simulink model "festo_proiect"  (R2022b)
settings: Solver=ode45  StartTime=0.0  StopTime=1500  RelTol=1e-3
undefined symbols (not defined in the file): A, C, dqi, hinitial, Hr, Hr1, Hr2, k, k1, k2, k3, k_comp, keta, qinitial, ua
libraries: slpidlib x7
(part 1 of 2)
settings Model: Creator=Alex  LastModifiedBy=Alex

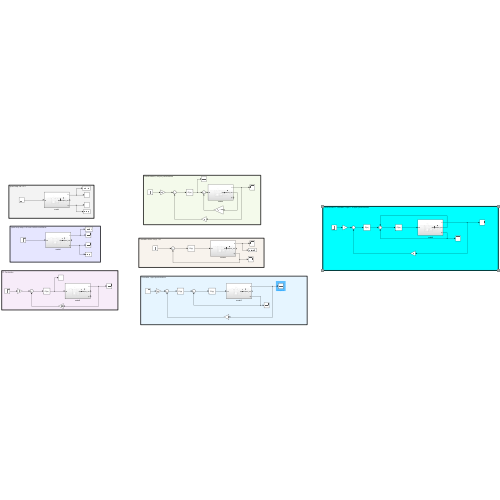
[thumbnail: Simulink's stored preview of the top-level diagram]
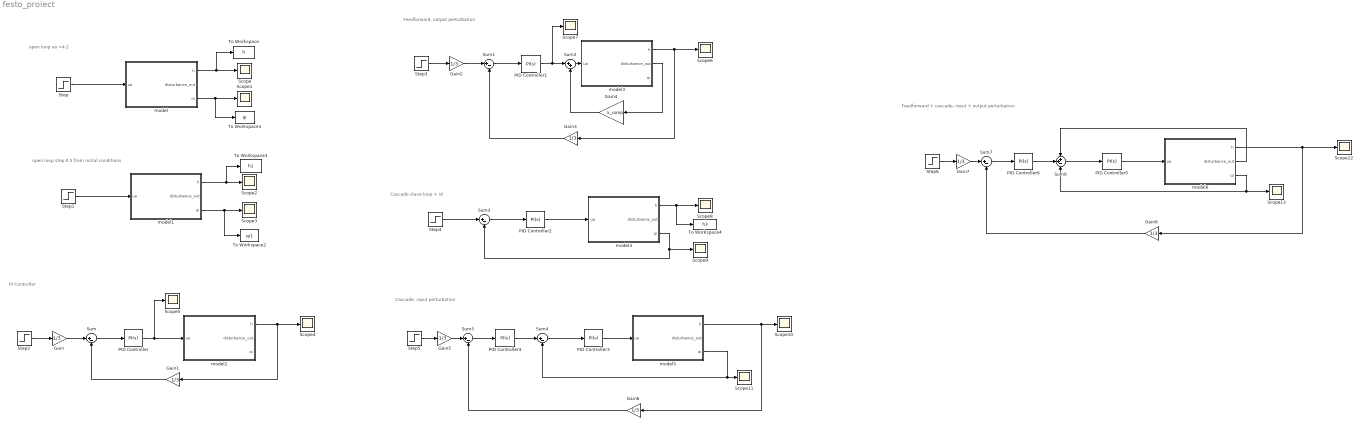
== system festo_proiect ==
  note: Feedforward + cascade, input + output perturbation
  note: Cascade, input perturbation
  note: Cascade slave loop + id
  note: Feedforward, output perturbation
  note: PI Controller
  note: open loop step 0.5 from initial conditions
  note: open loop ua =4.2
  Gain{,1..3,5..8} (8 alike) : Gain  Gain=1/3
  Gain4 : Gain  Gain=k_comp
  PID Controller : slpidlib/PID Controller  Controller=PI  Form=Parallel  TimeDomain=Continuous-time  UseExternalTs=off  SampleTime=-1  IntegratorMethod=Forward Euler  FilterMethod=Forward Euler  ControllerParametersSource=internal  P=Hr.Kp  I=Hr.kp/Hr.Ti  UseKiTs=off  D=0  N=100  UseFilter=on  TunerSelectOption=Transfer Function Based (PID Tuner App)  InitialConditionSource=internal  InitialConditionForIntegrator=ua  InitialConditionForFilter=0  DifferentiatorICPrevScaledInput=0  ExternalReset=none  TrackingMode=off  Kt=1  LimitOutput=off  SatLimitsSource=internal  UpperSaturationLimit=inf  LowerSaturationLimit=-inf  LinearizeAsGain=on  AntiWindupMode=none  Kb=1  LimitIntegrator=off  UpperIntegratorSaturationLimit=inf  LowerIntegratorSaturationLimit=-inf  POutMin=[]  POutMax=[]  IOutMin=[]  IOutMax=[]  DOutMin=[]  DOutMax=[]  NOutMin=[]  NOutMax=[]  SumOutMin=[]  SumOutMax=[]  SaturationOutMin=[]  SaturationOutMax=[]  PParamMin=[]  PParamMax=[]  IParamMin=[]  IParamMax=[]  DParamMin=[]  DParamMax=[]  NParamMin=[]  NParamMax=[]  KbParamMin=[]  KbParamMax=[]  KtParamMin=[]  KtParamMax=[]  KbOutMin=[]  KbOutMax=[]  KtOutMin=[]  KtOutMax=[]  IntegratorOutMin=[]  IntegratorOutMax=[]  FilterOutMin=[]  FilterOutMax=[]  SumI1OutMin=[]  SumI1OutMax=[]  SumI2OutMin=[]  SumI2OutMax=[]  SumI3OutMin=[]  SumI3OutMax=[]  SumI4OutMin=[]  SumI4OutMax=[]  SumDOutMin=[]  SumDOutMax=[]  DifferentiatorOutMin=[]  DifferentiatorOutMax=[]  FilterDiffOutCoefMin=[]  FilterDiffOutCoefMax=[]  ReciprocalOutMin=[]  ReciprocalOutMax=[]  SumDenOutMin=[]  SumDenOutMax=[]  SumNumOutMin=[]  SumNumOutMax=[]  DivideOutMin=[]  DivideOutMax=[]  UdiffTsProdOutMin=[]  UdiffTsProdOutMax=[]  NTsProdOutMin=[]  NTsProdOutMax=[]  UintegralTsProdOutMin=[]  UintegralTsProdOutMax=[]  UngainTsProdOutMin=[]  UngainTsProdOutMax=[]  ClampingZeroOutDataTypeStr=Inherit: Inherit via back propagation  ClampingZeroOutMin=[]  ClampingZeroOutMax=[]  FilterDenConstantOutDataTypeStr=Inherit: Inherit via back propagation  FilterDenConstantOutMin=[]  FilterDenConstantOutMax=[]  PCopyOutDataTypeStr=Inherit: Inherit via back propagation  PCopyOutMin=[]  PCopyOutMax=[]  NCopyOutDataTypeStr=Inherit: Inherit via back propagation  NCopyOutMin=[]  NCopyOutMax=[]  IntegratorContinuousStateAttributes=''  IntegratorStateMustResolveToSignalObject=off  IntegratorRTWStateStorageClass=Auto  FilterContinuousStateAttributes=''  FilterStateMustResolveToSignalObject=off  FilterRTWStateStorageClass=Auto  ParallelPVariant=InternalParameters  IdealPVariant=Disabled  IVariant=InternalParameters  DVariant=Disabled  IntegratorVariant=Continuous  SatVariant=Disabled  AWVariant=Passthrough  PCopyVariant=Disabled  TRVariant=Disabled  FdbkBlocksVariant=Forward  IdealPFdbkVariant=Disabled  SatFdbkVariant=Disabled  DerivativeFilterVariant=Disabled  NVariant=Disabled  NCopyVariant=Disabled_SignalSpec  FilterICVariant=Disabled  IntegratorICVariant=InternalICs  ExternalResetVariant=Disabled  TRSumVariant=Passthrough  SumFdbkVariant=Disabled  SumVariant=Sum_PI  TsampFilterVariant=InternalTs  TsampNgainVariant=Passthrough  TsampIntegralVariant=Passthrough  ExternalSaturationOutDataTypeStr=Inherit: Same as second input
  PID Controller1 : slpidlib/PID Controller  Controller=PI  Form=Parallel  TimeDomain=Continuous-time  UseExternalTs=off  SampleTime=-1  IntegratorMethod=Forward Euler  FilterMethod=Forward Euler  ControllerParametersSource=internal  P=Hr.Kp  I=Hr.kp/Hr.Ti  UseKiTs=off  D=0  N=100  UseFilter=on  TunerSelectOption=Transfer Function Based (PID Tuner App)  InitialConditionSource=internal  InitialConditionForIntegrator=ua  InitialConditionForFilter=0  DifferentiatorICPrevScaledInput=0  ExternalReset=none  TrackingMode=off  Kt=1  LimitOutput=off  SatLimitsSource=internal  UpperSaturationLimit=inf  LowerSaturationLimit=-inf  LinearizeAsGain=on  AntiWindupMode=none  Kb=1  LimitIntegrator=off  UpperIntegratorSaturationLimit=inf  LowerIntegratorSaturationLimit=-inf  POutMin=[]  POutMax=[]  IOutMin=[]  IOutMax=[]  DOutMin=[]  DOutMax=[]  NOutMin=[]  NOutMax=[]  SumOutMin=[]  SumOutMax=[]  SaturationOutMin=[]  SaturationOutMax=[]  PParamMin=[]  PParamMax=[]  IParamMin=[]  IParamMax=[]  DParamMin=[]  DParamMax=[]  NParamMin=[]  NParamMax=[]  KbParamMin=[]  KbParamMax=[]  KtParamMin=[]  KtParamMax=[]  KbOutMin=[]  KbOutMax=[]  KtOutMin=[]  KtOutMax=[]  IntegratorOutMin=[]  IntegratorOutMax=[]  FilterOutMin=[]  FilterOutMax=[]  SumI1OutMin=[]  SumI1OutMax=[]  SumI2OutMin=[]  SumI2OutMax=[]  SumI3OutMin=[]  SumI3OutMax=[]  SumI4OutMin=[]  SumI4OutMax=[]  SumDOutMin=[]  SumDOutMax=[]  DifferentiatorOutMin=[]  DifferentiatorOutMax=[]  FilterDiffOutCoefMin=[]  FilterDiffOutCoefMax=[]  ReciprocalOutMin=[]  ReciprocalOutMax=[]  SumDenOutMin=[]  SumDenOutMax=[]  SumNumOutMin=[]  SumNumOutMax=[]  DivideOutMin=[]  DivideOutMax=[]  UdiffTsProdOutMin=[]  UdiffTsProdOutMax=[]  NTsProdOutMin=[]  NTsProdOutMax=[]  UintegralTsProdOutMin=[]  UintegralTsProdOutMax=[]  UngainTsProdOutMin=[]  UngainTsProdOutMax=[]  ClampingZeroOutDataTypeStr=Inherit: Inherit via back propagation  ClampingZeroOutMin=[]  ClampingZeroOutMax=[]  FilterDenConstantOutDataTypeStr=Inherit: Inherit via back propagation  FilterDenConstantOutMin=[]  FilterDenConstantOutMax=[]  PCopyOutDataTypeStr=Inherit: Inherit via back propagation  PCopyOutMin=[]  PCopyOutMax=[]  NCopyOutDataTypeStr=Inherit: Inherit via back propagation  NCopyOutMin=[]  NCopyOutMax=[]  IntegratorContinuousStateAttributes=''  IntegratorStateMustResolveToSignalObject=off  IntegratorRTWStateStorageClass=Auto  FilterContinuousStateAttributes=''  FilterStateMustResolveToSignalObject=off  FilterRTWStateStorageClass=Auto  ParallelPVariant=InternalParameters  IdealPVariant=Disabled  IVariant=InternalParameters  DVariant=Disabled  IntegratorVariant=Continuous  SatVariant=Disabled  AWVariant=Passthrough  PCopyVariant=Disabled  TRVariant=Disabled  FdbkBlocksVariant=Forward  IdealPFdbkVariant=Disabled  SatFdbkVariant=Disabled  DerivativeFilterVariant=Disabled  NVariant=Disabled  NCopyVariant=Disabled_SignalSpec  FilterICVariant=Disabled  IntegratorICVariant=InternalICs  ExternalResetVariant=Disabled  TRSumVariant=Passthrough  SumFdbkVariant=Disabled  SumVariant=Sum_PI  TsampFilterVariant=InternalTs  TsampNgainVariant=Passthrough  TsampIntegralVariant=Passthrough  ExternalSaturationOutDataTypeStr=Inherit: Same as second input
  PID Controller2 : slpidlib/PID Controller  Controller=PI  Form=Parallel  TimeDomain=Continuous-time  UseExternalTs=off  SampleTime=-1  IntegratorMethod=Forward Euler  FilterMethod=Forward Euler  ControllerParametersSource=internal  P=Hr1.Kp  I=Hr1.Kp/Hr1.Ti  UseKiTs=off  D=0  N=100  UseFilter=on  TunerSelectOption=Transfer Function Based (PID Tuner App)  InitialConditionSource=internal  InitialConditionForIntegrator=ua  InitialConditionForFilter=0  DifferentiatorICPrevScaledInput=0  ExternalReset=none  TrackingMode=off  Kt=1  LimitOutput=off  SatLimitsSource=internal  UpperSaturationLimit=inf  LowerSaturationLimit=-inf  LinearizeAsGain=on  AntiWindupMode=none  Kb=1  LimitIntegrator=off  UpperIntegratorSaturationLimit=inf  LowerIntegratorSaturationLimit=-inf  POutMin=[]  POutMax=[]  IOutMin=[]  IOutMax=[]  DOutMin=[]  DOutMax=[]  NOutMin=[]  NOutMax=[]  SumOutMin=[]  SumOutMax=[]  SaturationOutMin=[]  SaturationOutMax=[]  PParamMin=[]  PParamMax=[]  IParamMin=[]  IParamMax=[]  DParamMin=[]  DParamMax=[]  NParamMin=[]  NParamMax=[]  KbParamMin=[]  KbParamMax=[]  KtParamMin=[]  KtParamMax=[]  KbOutMin=[]  KbOutMax=[]  KtOutMin=[]  KtOutMax=[]  IntegratorOutMin=[]  IntegratorOutMax=[]  FilterOutMin=[]  FilterOutMax=[]  SumI1OutMin=[]  SumI1OutMax=[]  SumI2OutMin=[]  SumI2OutMax=[]  SumI3OutMin=[]  SumI3OutMax=[]  SumI4OutMin=[]  SumI4OutMax=[]  SumDOutMin=[]  SumDOutMax=[]  DifferentiatorOutMin=[]  DifferentiatorOutMax=[]  FilterDiffOutCoefMin=[]  FilterDiffOutCoefMax=[]  ReciprocalOutMin=[]  ReciprocalOutMax=[]  SumDenOutMin=[]  SumDenOutMax=[]  SumNumOutMin=[]  SumNumOutMax=[]  DivideOutMin=[]  DivideOutMax=[]  UdiffTsProdOutMin=[]  UdiffTsProdOutMax=[]  NTsProdOutMin=[]  NTsProdOutMax=[]  UintegralTsProdOutMin=[]  UintegralTsProdOutMax=[]  UngainTsProdOutMin=[]  UngainTsProdOutMax=[]  ClampingZeroOutDataTypeStr=Inherit: Inherit via back propagation  ClampingZeroOutMin=[]  ClampingZeroOutMax=[]  FilterDenConstantOutDataTypeStr=Inherit: Inherit via back propagation  FilterDenConstantOutMin=[]  FilterDenConstantOutMax=[]  PCopyOutDataTypeStr=Inherit: Inherit via back propagation  PCopyOutMin=[]  PCopyOutMax=[]  NCopyOutDataTypeStr=Inherit: Inherit via back propagation  NCopyOutMin=[]  NCopyOutMax=[]  IntegratorContinuousStateAttributes=''  IntegratorStateMustResolveToSignalObject=off  IntegratorRTWStateStorageClass=Auto  FilterContinuousStateAttributes=''  FilterStateMustResolveToSignalObject=off  FilterRTWStateStorageClass=Auto  ParallelPVariant=InternalParameters  IdealPVariant=Disabled  IVariant=InternalParameters  DVariant=Disabled  IntegratorVariant=Continuous  SatVariant=Disabled  AWVariant=Passthrough  PCopyVariant=Disabled  TRVariant=Disabled  FdbkBlocksVariant=Forward  IdealPFdbkVariant=Disabled  SatFdbkVariant=Disabled  DerivativeFilterVariant=Disabled  NVariant=Disabled  NCopyVariant=Disabled_SignalSpec  FilterICVariant=Disabled  IntegratorICVariant=InternalICs  ExternalResetVariant=Disabled  TRSumVariant=Passthrough  SumFdbkVariant=Disabled  SumVariant=Sum_PI  TsampFilterVariant=InternalTs  TsampNgainVariant=Passthrough  TsampIntegralVariant=Passthrough  ExternalSaturationOutDataTypeStr=Inherit: Same as second input
  PID Controller3 : slpidlib/PID Controller  Controller=PI  Form=Parallel  TimeDomain=Continuous-time  UseExternalTs=off  SampleTime=-1  IntegratorMethod=Forward Euler  FilterMethod=Forward Euler  ControllerParametersSource=internal  P=Hr1.Kp  I=Hr1.Kp/Hr1.Ti  UseKiTs=off  D=0  N=100  UseFilter=on  TunerSelectOption=Transfer Function Based (PID Tuner App)  InitialConditionSource=internal  InitialConditionForIntegrator=ua  InitialConditionForFilter=0  DifferentiatorICPrevScaledInput=0  ExternalReset=none  TrackingMode=off  Kt=1  LimitOutput=off  SatLimitsSource=internal  UpperSaturationLimit=inf  LowerSaturationLimit=-inf  LinearizeAsGain=on  AntiWindupMode=none  Kb=1  LimitIntegrator=off  UpperIntegratorSaturationLimit=inf  LowerIntegratorSaturationLimit=-inf  POutMin=[]  POutMax=[]  IOutMin=[]  IOutMax=[]  DOutMin=[]  DOutMax=[]  NOutMin=[]  NOutMax=[]  SumOutMin=[]  SumOutMax=[]  SaturationOutMin=[]  SaturationOutMax=[]  PParamMin=[]  PParamMax=[]  IParamMin=[]  IParamMax=[]  DParamMin=[]  DParamMax=[]  NParamMin=[]  NParamMax=[]  KbParamMin=[]  KbParamMax=[]  KtParamMin=[]  KtParamMax=[]  KbOutMin=[]  KbOutMax=[]  KtOutMin=[]  KtOutMax=[]  IntegratorOutMin=[]  IntegratorOutMax=[]  FilterOutMin=[]  FilterOutMax=[]  SumI1OutMin=[]  SumI1OutMax=[]  SumI2OutMin=[]  SumI2OutMax=[]  SumI3OutMin=[]  SumI3OutMax=[]  SumI4OutMin=[]  SumI4OutMax=[]  SumDOutMin=[]  SumDOutMax=[]  DifferentiatorOutMin=[]  DifferentiatorOutMax=[]  FilterDiffOutCoefMin=[]  FilterDiffOutCoefMax=[]  ReciprocalOutMin=[]  ReciprocalOutMax=[]  SumDenOutMin=[]  SumDenOutMax=[]  SumNumOutMin=[]  SumNumOutMax=[]  DivideOutMin=[]  DivideOutMax=[]  UdiffTsProdOutMin=[]  UdiffTsProdOutMax=[]  NTsProdOutMin=[]  NTsProdOutMax=[]  UintegralTsProdOutMin=[]  UintegralTsProdOutMax=[]  UngainTsProdOutMin=[]  UngainTsProdOutMax=[]  ClampingZeroOutDataTypeStr=Inherit: Inherit via back propagation  ClampingZeroOutMin=[]  ClampingZeroOutMax=[]  FilterDenConstantOutDataTypeStr=Inherit: Inherit via back propagation  FilterDenConstantOutMin=[]  FilterDenConstantOutMax=[]  PCopyOutDataTypeStr=Inherit: Inherit via back propagation  PCopyOutMin=[]  PCopyOutMax=[]  NCopyOutDataTypeStr=Inherit: Inherit via back propagation  NCopyOutMin=[]  NCopyOutMax=[]  IntegratorContinuousStateAttributes=''  IntegratorStateMustResolveToSignalObject=off  IntegratorRTWStateStorageClass=Auto  FilterContinuousStateAttributes=''  FilterStateMustResolveToSignalObject=off  FilterRTWStateStorageClass=Auto  ParallelPVariant=InternalParameters  IdealPVariant=Disabled  IVariant=InternalParameters  DVariant=Disabled  IntegratorVariant=Continuous  SatVariant=Disabled  AWVariant=Passthrough  PCopyVariant=Disabled  TRVariant=Disabled  FdbkBlocksVariant=Forward  IdealPFdbkVariant=Disabled  SatFdbkVariant=Disabled  DerivativeFilterVariant=Disabled  NVariant=Disabled  NCopyVariant=Disabled_SignalSpec  FilterICVariant=Disabled  IntegratorICVariant=InternalICs  ExternalResetVariant=Disabled  TRSumVariant=Passthrough  SumFdbkVariant=Disabled  SumVariant=Sum_PI  TsampFilterVariant=InternalTs  TsampNgainVariant=Passthrough  TsampIntegralVariant=Passthrough  ExternalSaturationOutDataTypeStr=Inherit: Same as second input
  PID Controller4 : slpidlib/PID Controller  Controller=PI  Form=Parallel  TimeDomain=Continuous-time  UseExternalTs=off  SampleTime=-1  IntegratorMethod=Forward Euler  FilterMethod=Forward Euler  ControllerParametersSource=internal  P=Hr2.Kp  I=Hr2.Kp/Hr2.Ti  UseKiTs=off  D=0  N=100  UseFilter=on  TunerSelectOption=Transfer Function Based (PID Tuner App)  InitialConditionSource=internal  InitialConditionForIntegrator=qinitial  InitialConditionForFilter=0  DifferentiatorICPrevScaledInput=0  ExternalReset=none  TrackingMode=off  Kt=1  LimitOutput=off  SatLimitsSource=internal  UpperSaturationLimit=inf  LowerSaturationLimit=-inf  LinearizeAsGain=on  AntiWindupMode=none  Kb=1  LimitIntegrator=off  UpperIntegratorSaturationLimit=inf  LowerIntegratorSaturationLimit=-inf  POutMin=[]  POutMax=[]  IOutMin=[]  IOutMax=[]  DOutMin=[]  DOutMax=[]  NOutMin=[]  NOutMax=[]  SumOutMin=[]  SumOutMax=[]  SaturationOutMin=[]  SaturationOutMax=[]  PParamMin=[]  PParamMax=[]  IParamMin=[]  IParamMax=[]  DParamMin=[]  DParamMax=[]  NParamMin=[]  NParamMax=[]  KbParamMin=[]  KbParamMax=[]  KtParamMin=[]  KtParamMax=[]  KbOutMin=[]  KbOutMax=[]  KtOutMin=[]  KtOutMax=[]  IntegratorOutMin=[]  IntegratorOutMax=[]  FilterOutMin=[]  FilterOutMax=[]  SumI1OutMin=[]  SumI1OutMax=[]  SumI2OutMin=[]  SumI2OutMax=[]  SumI3OutMin=[]  SumI3OutMax=[]  SumI4OutMin=[]  SumI4OutMax=[]  SumDOutMin=[]  SumDOutMax=[]  DifferentiatorOutMin=[]  DifferentiatorOutMax=[]  FilterDiffOutCoefMin=[]  FilterDiffOutCoefMax=[]  ReciprocalOutMin=[]  ReciprocalOutMax=[]  SumDenOutMin=[]  SumDenOutMax=[]  SumNumOutMin=[]  SumNumOutMax=[]  DivideOutMin=[]  DivideOutMax=[]  UdiffTsProdOutMin=[]  UdiffTsProdOutMax=[]  NTsProdOutMin=[]  NTsProdOutMax=[]  UintegralTsProdOutMin=[]  UintegralTsProdOutMax=[]  UngainTsProdOutMin=[]  UngainTsProdOutMax=[]  ClampingZeroOutDataTypeStr=Inherit: Inherit via back propagation  ClampingZeroOutMin=[]  ClampingZeroOutMax=[]  FilterDenConstantOutDataTypeStr=Inherit: Inherit via back propagation  FilterDenConstantOutMin=[]  FilterDenConstantOutMax=[]  PCopyOutDataTypeStr=Inherit: Inherit via back propagation  PCopyOutMin=[]  PCopyOutMax=[]  NCopyOutDataTypeStr=Inherit: Inherit via back propagation  NCopyOutMin=[]  NCopyOutMax=[]  IntegratorContinuousStateAttributes=''  IntegratorStateMustResolveToSignalObject=off  IntegratorRTWStateStorageClass=Auto  FilterContinuousStateAttributes=''  FilterStateMustResolveToSignalObject=off  FilterRTWStateStorageClass=Auto  ParallelPVariant=InternalParameters  IdealPVariant=Disabled  IVariant=InternalParameters  DVariant=Disabled  IntegratorVariant=Continuous  SatVariant=Disabled  AWVariant=Passthrough  PCopyVariant=Disabled  TRVariant=Disabled  FdbkBlocksVariant=Forward  IdealPFdbkVariant=Disabled  SatFdbkVariant=Disabled  DerivativeFilterVariant=Disabled  NVariant=Disabled  NCopyVariant=Disabled_SignalSpec  FilterICVariant=Disabled  IntegratorICVariant=InternalICs  ExternalResetVariant=Disabled  TRSumVariant=Passthrough  SumFdbkVariant=Disabled  SumVariant=Sum_PI  TsampFilterVariant=InternalTs  TsampNgainVariant=Passthrough  TsampIntegralVariant=Passthrough  ExternalSaturationOutDataTypeStr=Inherit: Same as second input
  PID Controller5 : slpidlib/PID Controller  Controller=PI  Form=Parallel  TimeDomain=Continuous-time  UseExternalTs=off  SampleTime=-1  IntegratorMethod=Forward Euler  FilterMethod=Forward Euler  ControllerParametersSource=internal  P=Hr1.Kp  I=Hr1.Kp/Hr1.Ti  UseKiTs=off  D=0  N=100  UseFilter=on  TunerSelectOption=Transfer Function Based (PID Tuner App)  InitialConditionSource=internal  InitialConditionForIntegrator=ua  InitialConditionForFilter=0  DifferentiatorICPrevScaledInput=0  ExternalReset=none  TrackingMode=off  Kt=1  LimitOutput=off  SatLimitsSource=internal  UpperSaturationLimit=inf  LowerSaturationLimit=-inf  LinearizeAsGain=on  AntiWindupMode=none  Kb=1  LimitIntegrator=off  UpperIntegratorSaturationLimit=inf  LowerIntegratorSaturationLimit=-inf  POutMin=[]  POutMax=[]  IOutMin=[]  IOutMax=[]  DOutMin=[]  DOutMax=[]  NOutMin=[]  NOutMax=[]  SumOutMin=[]  SumOutMax=[]  SaturationOutMin=[]  SaturationOutMax=[]  PParamMin=[]  PParamMax=[]  IParamMin=[]  IParamMax=[]  DParamMin=[]  DParamMax=[]  NParamMin=[]  NParamMax=[]  KbParamMin=[]  KbParamMax=[]  KtParamMin=[]  KtParamMax=[]  KbOutMin=[]  KbOutMax=[]  KtOutMin=[]  KtOutMax=[]  IntegratorOutMin=[]  IntegratorOutMax=[]  FilterOutMin=[]  FilterOutMax=[]  SumI1OutMin=[]  SumI1OutMax=[]  SumI2OutMin=[]  SumI2OutMax=[]  SumI3OutMin=[]  SumI3OutMax=[]  SumI4OutMin=[]  SumI4OutMax=[]  SumDOutMin=[]  SumDOutMax=[]  DifferentiatorOutMin=[]  DifferentiatorOutMax=[]  FilterDiffOutCoefMin=[]  FilterDiffOutCoefMax=[]  ReciprocalOutMin=[]  ReciprocalOutMax=[]  SumDenOutMin=[]  SumDenOutMax=[]  SumNumOutMin=[]  SumNumOutMax=[]  DivideOutMin=[]  DivideOutMax=[]  UdiffTsProdOutMin=[]  UdiffTsProdOutMax=[]  NTsProdOutMin=[]  NTsProdOutMax=[]  UintegralTsProdOutMin=[]  UintegralTsProdOutMax=[]  UngainTsProdOutMin=[]  UngainTsProdOutMax=[]  ClampingZeroOutDataTypeStr=Inherit: Inherit via back propagation  ClampingZeroOutMin=[]  ClampingZeroOutMax=[]  FilterDenConstantOutDataTypeStr=Inherit: Inherit via back propagation  FilterDenConstantOutMin=[]  FilterDenConstantOutMax=[]  PCopyOutDataTypeStr=Inherit: Inherit via back propagation  PCopyOutMin=[]  PCopyOutMax=[]  NCopyOutDataTypeStr=Inherit: Inherit via back propagation  NCopyOutMin=[]  NCopyOutMax=[]  IntegratorContinuousStateAttributes=''  IntegratorStateMustResolveToSignalObject=off  IntegratorRTWStateStorageClass=Auto  FilterContinuousStateAttributes=''  FilterStateMustResolveToSignalObject=off  FilterRTWStateStorageClass=Auto  ParallelPVariant=InternalParameters  IdealPVariant=Disabled  IVariant=InternalParameters  DVariant=Disabled  IntegratorVariant=Continuous  SatVariant=Disabled  AWVariant=Passthrough  PCopyVariant=Disabled  TRVariant=Disabled  FdbkBlocksVariant=Forward  IdealPFdbkVariant=Disabled  SatFdbkVariant=Disabled  DerivativeFilterVariant=Disabled  NVariant=Disabled  NCopyVariant=Disabled_SignalSpec  FilterICVariant=Disabled  IntegratorICVariant=InternalICs  ExternalResetVariant=Disabled  TRSumVariant=Passthrough  SumFdbkVariant=Disabled  SumVariant=Sum_PI  TsampFilterVariant=InternalTs  TsampNgainVariant=Passthrough  TsampIntegralVariant=Passthrough  ExternalSaturationOutDataTypeStr=Inherit: Same as second input
  PID Controller6 : slpidlib/PID Controller  Controller=PI  Form=Parallel  TimeDomain=Continuous-time  UseExternalTs=off  SampleTime=-1  IntegratorMethod=Forward Euler  FilterMethod=Forward Euler  ControllerParametersSource=internal  P=Hr2.Kp  I=Hr2.Kp/Hr2.Ti  UseKiTs=off  D=0  N=100  UseFilter=on  TunerSelectOption=Transfer Function Based (PID Tuner App)  InitialConditionSource=internal  InitialConditionForIntegrator=qinitial  InitialConditionForFilter=0  DifferentiatorICPrevScaledInput=0  ExternalReset=none  TrackingMode=off  Kt=1  LimitOutput=off  SatLimitsSource=internal  UpperSaturationLimit=inf  LowerSaturationLimit=-inf  LinearizeAsGain=on  AntiWindupMode=none  Kb=1  LimitIntegrator=off  UpperIntegratorSaturationLimit=inf  LowerIntegratorSaturationLimit=-inf  POutMin=[]  POutMax=[]  IOutMin=[]  IOutMax=[]  DOutMin=[]  DOutMax=[]  NOutMin=[]  NOutMax=[]  SumOutMin=[]  SumOutMax=[]  SaturationOutMin=[]  SaturationOutMax=[]  PParamMin=[]  PParamMax=[]  IParamMin=[]  IParamMax=[]  DParamMin=[]  DParamMax=[]  NParamMin=[]  NParamMax=[]  KbParamMin=[]  KbParamMax=[]  KtParamMin=[]  KtParamMax=[]  KbOutMin=[]  KbOutMax=[]  KtOutMin=[]  KtOutMax=[]  IntegratorOutMin=[]  IntegratorOutMax=[]  FilterOutMin=[]  FilterOutMax=[]  SumI1OutMin=[]  SumI1OutMax=[]  SumI2OutMin=[]  SumI2OutMax=[]  SumI3OutMin=[]  SumI3OutMax=[]  SumI4OutMin=[]  SumI4OutMax=[]  SumDOutMin=[]  SumDOutMax=[]  DifferentiatorOutMin=[]  DifferentiatorOutMax=[]  FilterDiffOutCoefMin=[]  FilterDiffOutCoefMax=[]  ReciprocalOutMin=[]  ReciprocalOutMax=[]  SumDenOutMin=[]  SumDenOutMax=[]  SumNumOutMin=[]  SumNumOutMax=[]  DivideOutMin=[]  DivideOutMax=[]  UdiffTsProdOutMin=[]  UdiffTsProdOutMax=[]  NTsProdOutMin=[]  NTsProdOutMax=[]  UintegralTsProdOutMin=[]  UintegralTsProdOutMax=[]  UngainTsProdOutMin=[]  UngainTsProdOutMax=[]  ClampingZeroOutDataTypeStr=Inherit: Inherit via back propagation  ClampingZeroOutMin=[]  ClampingZeroOutMax=[]  FilterDenConstantOutDataTypeStr=Inherit: Inherit via back propagation  FilterDenConstantOutMin=[]  FilterDenConstantOutMax=[]  PCopyOutDataTypeStr=Inherit: Inherit via back propagation  PCopyOutMin=[]  PCopyOutMax=[]  NCopyOutDataTypeStr=Inherit: Inherit via back propagation  NCopyOutMin=[]  NCopyOutMax=[]  IntegratorContinuousStateAttributes=''  IntegratorStateMustResolveToSignalObject=off  IntegratorRTWStateStorageClass=Auto  FilterContinuousStateAttributes=''  FilterStateMustResolveToSignalObject=off  FilterRTWStateStorageClass=Auto  ParallelPVariant=InternalParameters  IdealPVariant=Disabled  IVariant=InternalParameters  DVariant=Disabled  IntegratorVariant=Continuous  SatVariant=Disabled  AWVariant=Passthrough  PCopyVariant=Disabled  TRVariant=Disabled  FdbkBlocksVariant=Forward  IdealPFdbkVariant=Disabled  SatFdbkVariant=Disabled  DerivativeFilterVariant=Disabled  NVariant=Disabled  NCopyVariant=Disabled_SignalSpec  FilterICVariant=Disabled  IntegratorICVariant=InternalICs  ExternalResetVariant=Disabled  TRSumVariant=Passthrough  SumFdbkVariant=Disabled  SumVariant=Sum_PI  TsampFilterVariant=InternalTs  TsampNgainVariant=Passthrough  TsampIntegralVariant=Passthrough  ExternalSaturationOutDataTypeStr=Inherit: Same as second input
  Scope{,1..13} (14 alike) : Scope
  Step : Step  Time=0  After=ua  SampleTime=0
  Step1 : Step  Time=0  Before=ua  After=ua+0.5  SampleTime=0
  Step{2..3,5..6} (4 alike) : Step  Time=0  Before=hinitial  After=13  SampleTime=0
  Step4 : Step  Time=0  Before=qinitial  After=qinitial+dqi  SampleTime=0
  Sum{,1,3..5,7} (6 alike) : Sum  Inputs=|+-
  Sum2 : Sum  Inputs=|++
  Sum6 : Sum  Inputs=++-
  To Workspace : ToWorkspace  VariableName=h  SampleTime=-1
  To Workspace1 : ToWorkspace  VariableName=qi  SampleTime=-1
  To Workspace2 : ToWorkspace  VariableName=qi1  SampleTime=-1
  To Workspace3 : ToWorkspace  VariableName=h1  SampleTime=-1
  To Workspace4 : ToWorkspace  VariableName=h3  SampleTime=-1
  model : Subsystem
  model1 : Subsystem
  model2 : Subsystem
  model3 : Subsystem
  model4 : Subsystem
  model5 : Subsystem
  model6 : Subsystem
  wires:
  Step/1 -> model/1(ua)
  model/1(h) -> To Workspace/1, Scope/1
  model/3(qi) -> To Workspace1/1, Scope1/1
  Step1/1 -> model1/1(ua)
  model1/3(qi) -> To Workspace2/1, Scope3/1
  model1/1(h) -> To Workspace3/1, Scope2/1
  model2/1(h) -> Scope4/1, Gain1/1
  PID Controller/1 -> Scope5/1, model2/1(ua)
  Sum/1 -> PID Controller/1
  Gain/1 -> Sum/1
  Step2/1 -> Gain/1
  Gain1/1 -> Sum/2
  Gain3/1 -> Sum1/2
  Step3/1 -> Gain2/1
  Gain2/1 -> Sum1/1
  Sum1/1 -> PID Controller1/1
  PID Controller1/1 -> Sum2/1, Scope7/1
  model3/1(h) -> Gain3/1, Scope6/1
  Sum2/1 -> model3/1(ua)
  model3/2(disturbance_out) -> Gain4/1
  Gain4/1 -> Sum2/2
  model4/1(h) -> To Workspace4/1, Scope8/1
  PID Controller2/1 -> model4/1(ua)
  Sum3/1 -> PID Controller2/1
  model4/3(qi) -> Scope9/1, Sum3/2
  Step4/1 -> Sum3/1
  model5/3(qi) -> Sum4/2, Scope11/1
  Sum4/1 -> PID Controller3/1
  PID Controller3/1 -> model5/1(ua)
  model5/1(h) -> Scope10/1, Gain6/1
  PID Controller4/1 -> Sum4/1
  Step5/1 -> Gain5/1
  Sum5/1 -> PID Controller4/1
  Gain5/1 -> Sum5/1
  Gain6/1 -> Sum5/2
  Gain8/1 -> Sum7/2
  Gain7/1 -> Sum7/1
  Sum7/1 -> PID Controller6/1
  Step6/1 -> Gain7/1
  PID Controller6/1 -> Sum6/2
  model6/1(h) -> Gain8/1, Scope12/1
  PID Controller5/1 -> model6/1(ua)
  Sum6/1 -> PID Controller5/1
  model6/3(qi) -> Sum6/3, Scope13/1
  model6/2(disturbance_out) -> Sum6/1

== system festo_proiect/model ==
  ua : Inport
  Amplificator : Subsystem
  Curent rotoric : Subsystem
  Filtru : Subsystem
  Motor : Subsystem
  Pompa : Subsystem
  Randament pompa : Subsystem
  Rezervor : Subsystem
  disturbance_in : Step  Commented=on  Time=250  After=0.1*k  SampleTime=0
  h : Outport
  disturbance_out : Outport  Port=2
  qi : Outport  Port=3
  wires:
  Randament pompa/1(eta) -> Curent rotoric/2(eta)
  Rezervor/1(h) -> h/1, Pompa/2(h), Curent rotoric/3(h)
  Amplificator/1(um) -> Curent rotoric/4(um), Randament pompa/2(um), Motor/1(um)
  Motor/1(km*n) -> Pompa/1(km*n)
  ua/1 -> Amplificator/1(ua)
  Curent rotoric/1(im) -> Motor/2(im)
  Pompa/1(q) -> Filtru/1(q)
  Filtru/1(q_f) -> Rezervor/1(q), qi/1, Curent rotoric/1(q), Randament pompa/1(q)
  disturbance_in/1 -> Pompa/3(perturbatie k)
  Rezervor/2(disturbance_out) -> disturbance_out/1

== system festo_proiect/model1 ==
  ua : Inport
  Amplificator : Subsystem
  Curent rotoric : Subsystem
  Filtru : Subsystem
  Motor : Subsystem
  Pompa : Subsystem
  Randament pompa : Subsystem
  Rezervor : Subsystem
  disturbance_in : Step  Commented=on  Time=250  After=0.1*k  SampleTime=0
  h : Outport
  disturbance_out : Outport  Port=2
  qi : Outport  Port=3
  wires:
  Rezervor/2(disturbance_out) -> disturbance_out/1
  disturbance_in/1 -> Pompa/3(perturbatie k)
  Filtru/1(q_f) -> Randament pompa/1(q), Curent rotoric/1(q), qi/1, Rezervor/1(q)
  Pompa/1(q) -> Filtru/1(q)
  Curent rotoric/1(im) -> Motor/2(im)
  ua/1 -> Amplificator/1(ua)
  Motor/1(km*n) -> Pompa/1(km*n)
  Amplificator/1(um) -> Motor/1(um), Randament pompa/2(um), Curent rotoric/4(um)
  Rezervor/1(h) -> Curent rotoric/3(h), Pompa/2(h), h/1
  Randament pompa/1(eta) -> Curent rotoric/2(eta)

== system festo_proiect/model2 ==
  ua : Inport
  Amplificator : Subsystem
  Curent rotoric : Subsystem
  Filtru : Subsystem
  Motor : Subsystem
  Pompa : Subsystem
  Randament pompa : Subsystem
  Rezervor : Subsystem
  disturbance_in : Step  Commented=on  Time=250  After=0.1*k  SampleTime=0
  h : Outport
  disturbance_out : Outport  Port=2
  qi : Outport  Port=3
  wires:
  Randament pompa/1(eta) -> Curent rotoric/2(eta)
  Rezervor/1(h) -> h/1, Pompa/2(h), Curent rotoric/3(h)
  Amplificator/1(um) -> Curent rotoric/4(um), Randament pompa/2(um), Motor/1(um)
  Motor/1(km*n) -> Pompa/1(km*n)
  ua/1 -> Amplificator/1(ua)
  Curent rotoric/1(im) -> Motor/2(im)
  Pompa/1(q) -> Filtru/1(q)
  Filtru/1(q_f) -> Rezervor/1(q), qi/1, Curent rotoric/1(q), Randament pompa/1(q)
  disturbance_in/1 -> Pompa/3(perturbatie k)
  Rezervor/2(disturbance_out) -> disturbance_out/1

== system festo_proiect/model3 ==
  ua : Inport
  Amplificator : Subsystem
  Curent rotoric : Subsystem
  Filtru : Subsystem
  Motor : Subsystem
  Pompa : Subsystem
  Randament pompa : Subsystem
  Rezervor : Subsystem
  disturbance_in : Step  Commented=on  Time=250  After=0.1*k  SampleTime=0
  h : Outport
  disturbance_out : Outport  Port=2
  qi : Outport  Port=3
  wires:
  Rezervor/2(disturbance_out) -> disturbance_out/1
  disturbance_in/1 -> Pompa/3(perturbatie k)
  Filtru/1(q_f) -> Randament pompa/1(q), Curent rotoric/1(q), qi/1, Rezervor/1(q)
  Pompa/1(q) -> Filtru/1(q)
  Curent rotoric/1(im) -> Motor/2(im)
  ua/1 -> Amplificator/1(ua)
  Motor/1(km*n) -> Pompa/1(km*n)
  Amplificator/1(um) -> Motor/1(um), Randament pompa/2(um), Curent rotoric/4(um)
  Rezervor/1(h) -> Curent rotoric/3(h), Pompa/2(h), h/1
  Randament pompa/1(eta) -> Curent rotoric/2(eta)

== system festo_proiect/model4 ==
  ua : Inport
  Amplificator : Subsystem
  Curent rotoric : Subsystem
  Filtru : Subsystem
  Motor : Subsystem
  Pompa : Subsystem
  Randament pompa : Subsystem
  Rezervor : Subsystem
  disturbance_in : Step  Commented=on  Time=250  After=0.1*k  SampleTime=0
  h : Outport
  disturbance_out : Outport  Port=2
  qi : Outport  Port=3
  wires:
  Randament pompa/1(eta) -> Curent rotoric/2(eta)
  Rezervor/1(h) -> h/1, Pompa/2(h), Curent rotoric/3(h)
  Amplificator/1(um) -> Curent rotoric/4(um), Randament pompa/2(um), Motor/1(um)
  Motor/1(km*n) -> Pompa/1(km*n)
  ua/1 -> Amplificator/1(ua)
  Curent rotoric/1(im) -> Motor/2(im)
  Pompa/1(q) -> Filtru/1(q)
  Filtru/1(q_f) -> Rezervor/1(q), qi/1, Curent rotoric/1(q), Randament pompa/1(q)
  disturbance_in/1 -> Pompa/3(perturbatie k)
  Rezervor/2(disturbance_out) -> disturbance_out/1

== system festo_proiect/model5 ==
  ua : Inport
  Amplificator : Subsystem
  Curent rotoric : Subsystem
  Filtru : Subsystem
  Motor : Subsystem
  Pompa : Subsystem
  Randament pompa : Subsystem
  Rezervor : Subsystem
  disturbance_in : Step  Time=250  After=0.1*k  SampleTime=0
  h : Outport
  disturbance_out : Outport  Port=2
  qi : Outport  Port=3
  wires:
  Rezervor/2(disturbance_out) -> disturbance_out/1
  disturbance_in/1 -> Pompa/3(perturbatie k)
  Filtru/1(q_f) -> Randament pompa/1(q), Curent rotoric/1(q), qi/1, Rezervor/1(q)
  Pompa/1(q) -> Filtru/1(q)
  Curent rotoric/1(im) -> Motor/2(im)
  ua/1 -> Amplificator/1(ua)
  Motor/1(km*n) -> Pompa/1(km*n)
  Amplificator/1(um) -> Motor/1(um), Randament pompa/2(um), Curent rotoric/4(um)
  Rezervor/1(h) -> Curent rotoric/3(h), Pompa/2(h), h/1
  Randament pompa/1(eta) -> Curent rotoric/2(eta)

== system festo_proiect/model6 ==
  ua : Inport
  Amplificator : Subsystem
  Curent rotoric : Subsystem
  Filtru : Subsystem
  Motor : Subsystem
  Pompa : Subsystem
  Randament pompa : Subsystem
  Rezervor : Subsystem
  disturbance_in : Step  Time=250  After=0.1*k  SampleTime=0
  h : Outport
  disturbance_out : Outport  Port=2
  qi : Outport  Port=3
  wires:
  Randament pompa/1(eta) -> Curent rotoric/2(eta)
  Rezervor/1(h) -> h/1, Pompa/2(h), Curent rotoric/3(h)
  Amplificator/1(um) -> Curent rotoric/4(um), Randament pompa/2(um), Motor/1(um)
  Motor/1(km*n) -> Pompa/1(km*n)
  ua/1 -> Amplificator/1(ua)
  Curent rotoric/1(im) -> Motor/2(im)
  Pompa/1(q) -> Filtru/1(q)
  Filtru/1(q_f) -> Rezervor/1(q), qi/1, Curent rotoric/1(q), Randament pompa/1(q)
  disturbance_in/1 -> Pompa/3(perturbatie k)
  Rezervor/2(disturbance_out) -> disturbance_out/1

== system festo_proiect/model/Amplificator ==
  ua : Inport
  Constant : Constant  Value=8.1
  Gain : Gain  Gain=2.2
  Gain1 : Gain  Gain=2.2
  Gain2 : Gain  Gain=5
  Saturation : Saturate  UpperLimit=22  LowerLimit=0
  Sum : Sum  Inputs=|++
  Sum1 : Sum  Inputs=|+-
  Switch : Switch  Threshold=8.1  SaturateOnIntegerOverflow=off  InputSameDT=off
  um : Outport
  wires:
  ua/1 -> Switch/2, Gain/1, Sum1/1, Gain1/1
  Gain1/1 -> Sum/1
  Constant/1 -> Sum1/2
  Sum1/1 -> Gain2/1
  Gain2/1 -> Sum/2
  Switch/1 -> Saturation/1
  Saturation/1 -> um/1
  Gain/1 -> Switch/3
  Sum/1 -> Switch/1

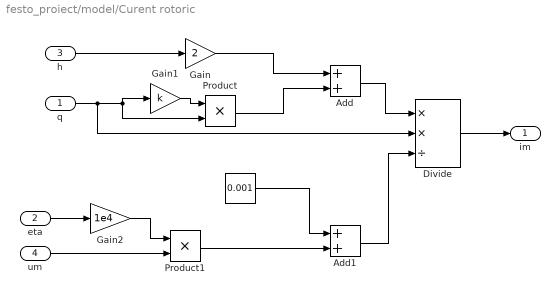
== system festo_proiect/model/Curent rotoric ==
  q : Inport
  eta : Inport  Port=2
  h : Inport  Port=3
  um : Inport  Port=4
  "  " : Constant  Value=0.001
  Add : Sum
  Add1 : Sum
  Divide : Product  Inputs=**/
  Gain : Gain  Gain=2
  Gain1 : Gain  Gain=k
  Gain2 : Gain  Gain=1e4
  Product : Product
  Product1 : Product
  im : Outport
  wires:
  h/1 -> Gain/1
  q/1 -> Divide/2, Gain1/1, Product/2
  Gain/1 -> Add/1
  Product/1 -> Add/2
  um/1 -> Product1/2
  "  "/1 -> Add1/1
  Product1/1 -> Add1/2
  Add/1 -> Divide/1
  Add1/1 -> Divide/3
  Divide/1 -> im/1
  eta/1 -> Gain2/1
  Gain2/1 -> Product1/1
  Gain1/1 -> Product/1

== system festo_proiect/model/Filtru ==
  q : Inport
  Integrator : Integrator
  Sum : Sum  Inputs=|+-
  q_f : Outport
  wires:
  q/1 -> Sum/1
  Sum/1 -> Integrator/1
  Integrator/1 -> Sum/2, q_f/1

== system festo_proiect/model/Motor ==
  um : Inport
  im : Inport  Port=2
  Add : Sum  Inputs=+-
  Rm : Gain  Gain=3
  km*n : Outport
  wires:
  um/1 -> Add/1
  im/1 -> Rm/1
  Rm/1 -> Add/2
  Add/1 -> km*n/1

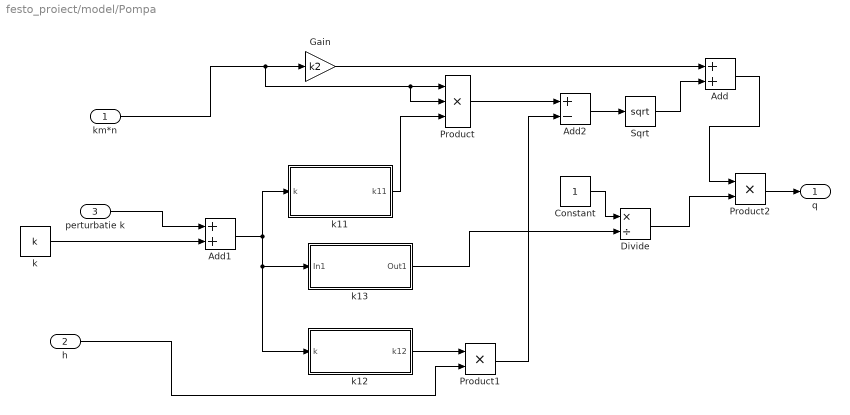
== system festo_proiect/model/Pompa ==
  km*n : Inport
  h : Inport  Port=2
  perturbatie k : Inport  Port=3
  Add : Sum
  Add1 : Sum
  Add2 : Sum  Inputs=+-
  Constant : Constant
  Divide : Product  Inputs=*/
  Gain : Gain  Gain=k2
  Product : Product  Inputs=3
  Product1 : Product
  Product2 : Product
  Sqrt : Sqrt
  k : Constant  Value=k
  k11 : Subsystem
  k12 : Subsystem
  k13 : Subsystem
  q : Outport
  wires:
  km*n/1 -> Product/2, Product/1, Gain/1
  perturbatie k/1 -> Add1/1
  k/1 -> Add1/2
  Add1/1 -> k11/1(k), k12/1(k), k13/1(In1)
  k11/1(k11) -> Product/3
  Gain/1 -> Add/1
  Product/1 -> Add2/1
  h/1 -> Product1/2
  k12/1(k12) -> Product1/1
  Product1/1 -> Add2/2
  Add2/1 -> Sqrt/1
  Sqrt/1 -> Add/2
  Add/1 -> Product2/1
  k13/1(Out1) -> Divide/2
  Constant/1 -> Divide/1
  Divide/1 -> Product2/2
  Product2/1 -> q/1

== system festo_proiect/model/Randament pompa ==
  q : Inport
  um : Inport  Port=2
  Gain : Gain  Gain=keta
  Product : Product
  eta : Outport
  wires:
  um/1 -> Gain/1
  q/1 -> Product/1
  Gain/1 -> Product/2
  Product/1 -> eta/1

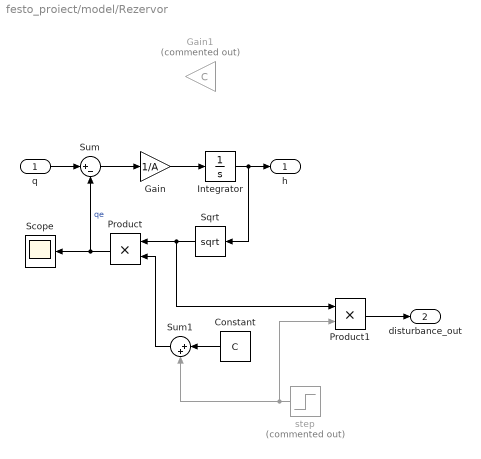
== system festo_proiect/model/Rezervor ==
  q : Inport
  Constant : Constant  Value=C
  Gain : Gain  Gain=1/A
  Gain1 : Gain  Commented=on  Gain=C
  Integrator : Integrator
  Product : Product
  Product1 : Product
  Scope : Scope
  Sqrt : Sqrt
  Sum : Sum  Inputs=|+-
  Sum1 : Sum  Inputs=|++
  step : Step  Commented=on  Time=300  After=0  SampleTime=0
  h : Outport
  disturbance_out : Outport  Port=2
  wires:
  q/1 -> Sum/1
  Sum/1 -> Gain/1
  Gain/1 -> Integrator/1
  Integrator/1 -> Sqrt/1, h/1
  Sqrt/1 -> Product1/1, Product/1
  Product/1 -> Sum/2, Scope/1  "qe"
  step/1 -> Sum1/2, Product1/2
  Constant/1 -> Sum1/1
  Sum1/1 -> Product/2
  Product1/1 -> disturbance_out/1

== system festo_proiect/model1/Amplificator ==
  ua : Inport
  Constant : Constant  Value=8.1
  Gain : Gain  Gain=2.2
  Gain1 : Gain  Gain=2.2
  Gain2 : Gain  Gain=5
  Saturation : Saturate  UpperLimit=22  LowerLimit=0
  Sum : Sum  Inputs=|++
  Sum1 : Sum  Inputs=|+-
  Switch : Switch  Threshold=8.1  SaturateOnIntegerOverflow=off  InputSameDT=off
  um : Outport
  wires:
  Sum/1 -> Switch/1
  Gain/1 -> Switch/3
  Saturation/1 -> um/1
  Switch/1 -> Saturation/1
  Gain2/1 -> Sum/2
  Sum1/1 -> Gain2/1
  Constant/1 -> Sum1/2
  Gain1/1 -> Sum/1
  ua/1 -> Gain1/1, Sum1/1, Gain/1, Switch/2

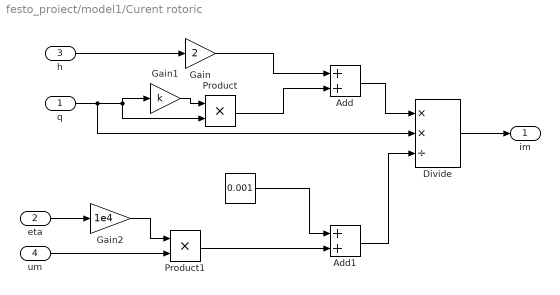
== system festo_proiect/model1/Curent rotoric ==
  q : Inport
  eta : Inport  Port=2
  h : Inport  Port=3
  um : Inport  Port=4
  "  " : Constant  Value=0.001
  Add : Sum
  Add1 : Sum
  Divide : Product  Inputs=**/
  Gain : Gain  Gain=2
  Gain1 : Gain  Gain=k
  Gain2 : Gain  Gain=1e4
  Product : Product
  Product1 : Product
  im : Outport
  wires:
  Gain1/1 -> Product/1
  Gain2/1 -> Product1/1
  eta/1 -> Gain2/1
  Divide/1 -> im/1
  Add1/1 -> Divide/3
  Add/1 -> Divide/1
  Product1/1 -> Add1/2
  "  "/1 -> Add1/1
  um/1 -> Product1/2
  Product/1 -> Add/2
  Gain/1 -> Add/1
  q/1 -> Product/2, Gain1/1, Divide/2
  h/1 -> Gain/1

== system festo_proiect/model1/Filtru ==
  q : Inport
  Integrator : Integrator  InitialCondition=qinitial
  Sum : Sum  Inputs=|+-
  q_f : Outport
  wires:
  Integrator/1 -> q_f/1, Sum/2
  Sum/1 -> Integrator/1
  q/1 -> Sum/1

== system festo_proiect/model1/Motor ==
  um : Inport
  im : Inport  Port=2
  Add : Sum  Inputs=+-
  Rm : Gain  Gain=3
  km*n : Outport
  wires:
  Add/1 -> km*n/1
  Rm/1 -> Add/2
  im/1 -> Rm/1
  um/1 -> Add/1

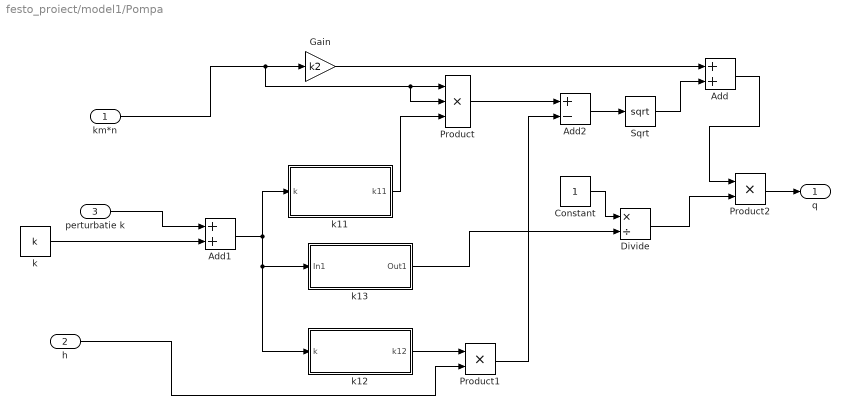
== system festo_proiect/model1/Pompa ==
  km*n : Inport
  h : Inport  Port=2
  perturbatie k : Inport  Port=3
  Add : Sum
  Add1 : Sum
  Add2 : Sum  Inputs=+-
  Constant : Constant
  Divide : Product  Inputs=*/
  Gain : Gain  Gain=k2
  Product : Product  Inputs=3
  Product1 : Product
  Product2 : Product
  Sqrt : Sqrt
  k : Constant  Value=k
  k11 : Subsystem
  k12 : Subsystem
  k13 : Subsystem
  q : Outport
  wires:
  Product2/1 -> q/1
  Divide/1 -> Product2/2
  Constant/1 -> Divide/1
  k13/1(Out1) -> Divide/2
  Add/1 -> Product2/1
  Sqrt/1 -> Add/2
  Add2/1 -> Sqrt/1
  Product1/1 -> Add2/2
  k12/1(k12) -> Product1/1
  h/1 -> Product1/2
  Product/1 -> Add2/1
  Gain/1 -> Add/1
  k11/1(k11) -> Product/3
  Add1/1 -> k13/1(In1), k12/1(k), k11/1(k)
  k/1 -> Add1/2
  perturbatie k/1 -> Add1/1
  km*n/1 -> Gain/1, Product/1, Product/2

== system festo_proiect/model1/Randament pompa ==
  q : Inport
  um : Inport  Port=2
  Gain : Gain  Gain=keta
  Product : Product
  eta : Outport
  wires:
  Product/1 -> eta/1
  Gain/1 -> Product/2
  q/1 -> Product/1
  um/1 -> Gain/1

== system festo_proiect/model1/Rezervor ==
  q : Inport
  Constant : Constant  Value=C
  Gain : Gain  Gain=1/A
  Integrator : Integrator  InitialCondition=hinitial
  Product : Product
  Product1 : Product
  Scope : Scope
  Sqrt : Sqrt
  Sum : Sum  Inputs=|+-
  Sum1 : Sum  Inputs=|++
  step : Step  Commented=on  Time=300  After=0  SampleTime=0
  h : Outport
  disturbance_out : Outport  Port=2
  wires:
  Product1/1 -> disturbance_out/1
  Sum1/1 -> Product/2
  Constant/1 -> Sum1/1
  step/1 -> Product1/2, Sum1/2
  Product/1 -> Scope/1, Sum/2  "qe"
  Sqrt/1 -> Product/1, Product1/1
  Integrator/1 -> h/1, Sqrt/1
  Gain/1 -> Integrator/1
  Sum/1 -> Gain/1
  q/1 -> Sum/1

== system festo_proiect/model2/Amplificator ==
  ua : Inport
  Constant : Constant  Value=8.1
  Gain : Gain  Gain=2.2
  Gain1 : Gain  Gain=2.2
  Gain2 : Gain  Gain=5
  Saturation : Saturate  UpperLimit=22  LowerLimit=0
  Sum : Sum  Inputs=|++
  Sum1 : Sum  Inputs=|+-
  Switch : Switch  Threshold=8.1  SaturateOnIntegerOverflow=off  InputSameDT=off
  um : Outport
  wires:
  ua/1 -> Switch/2, Gain/1, Sum1/1, Gain1/1
  Gain1/1 -> Sum/1
  Constant/1 -> Sum1/2
  Sum1/1 -> Gain2/1
  Gain2/1 -> Sum/2
  Switch/1 -> Saturation/1
  Saturation/1 -> um/1
  Gain/1 -> Switch/3
  Sum/1 -> Switch/1

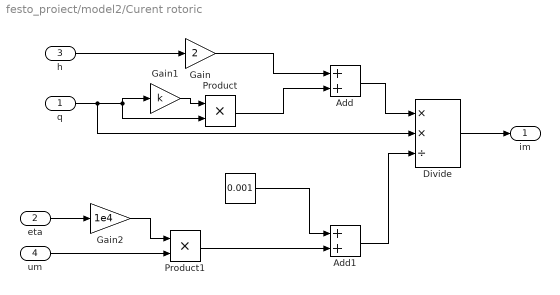
== system festo_proiect/model2/Curent rotoric ==
  q : Inport
  eta : Inport  Port=2
  h : Inport  Port=3
  um : Inport  Port=4
  "  " : Constant  Value=0.001
  Add : Sum
  Add1 : Sum
  Divide : Product  Inputs=**/
  Gain : Gain  Gain=2
  Gain1 : Gain  Gain=k
  Gain2 : Gain  Gain=1e4
  Product : Product
  Product1 : Product
  im : Outport
  wires:
  h/1 -> Gain/1
  q/1 -> Divide/2, Gain1/1, Product/2
  Gain/1 -> Add/1
  Product/1 -> Add/2
  um/1 -> Product1/2
  "  "/1 -> Add1/1
  Product1/1 -> Add1/2
  Add/1 -> Divide/1
  Add1/1 -> Divide/3
  Divide/1 -> im/1
  eta/1 -> Gain2/1
  Gain2/1 -> Product1/1
  Gain1/1 -> Product/1

== system festo_proiect/model2/Filtru ==
  q : Inport
  Integrator : Integrator  InitialCondition=qinitial
  Sum : Sum  Inputs=|+-
  q_f : Outport
  wires:
  q/1 -> Sum/1
  Sum/1 -> Integrator/1
  Integrator/1 -> Sum/2, q_f/1

== system festo_proiect/model2/Motor ==
  um : Inport
  im : Inport  Port=2
  Add : Sum  Inputs=+-
  Rm : Gain  Gain=3
  km*n : Outport
  wires:
  um/1 -> Add/1
  im/1 -> Rm/1
  Rm/1 -> Add/2
  Add/1 -> km*n/1

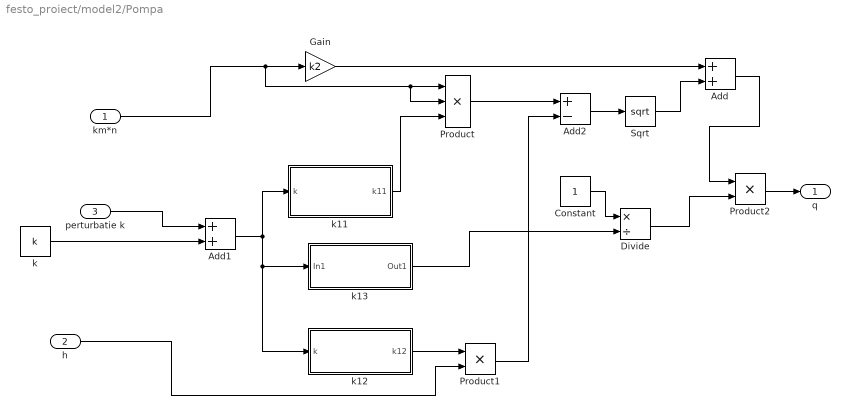
== system festo_proiect/model2/Pompa ==
  km*n : Inport
  h : Inport  Port=2
  perturbatie k : Inport  Port=3
  Add : Sum
  Add1 : Sum
  Add2 : Sum  Inputs=+-
  Constant : Constant
  Divide : Product  Inputs=*/
  Gain : Gain  Gain=k2
  Product : Product  Inputs=3
  Product1 : Product
  Product2 : Product
  Sqrt : Sqrt
  k : Constant  Value=k
  k11 : Subsystem
  k12 : Subsystem
  k13 : Subsystem
  q : Outport
  wires:
  km*n/1 -> Product/2, Product/1, Gain/1
  perturbatie k/1 -> Add1/1
  k/1 -> Add1/2
  Add1/1 -> k11/1(k), k12/1(k), k13/1(In1)
  k11/1(k11) -> Product/3
  Gain/1 -> Add/1
  Product/1 -> Add2/1
  h/1 -> Product1/2
  k12/1(k12) -> Product1/1
  Product1/1 -> Add2/2
  Add2/1 -> Sqrt/1
  Sqrt/1 -> Add/2
  Add/1 -> Product2/1
  k13/1(Out1) -> Divide/2
  Constant/1 -> Divide/1
  Divide/1 -> Product2/2
  Product2/1 -> q/1

== system festo_proiect/model2/Randament pompa ==
  q : Inport
  um : Inport  Port=2
  Gain : Gain  Gain=keta
  Product : Product
  eta : Outport
  wires:
  um/1 -> Gain/1
  q/1 -> Product/1
  Gain/1 -> Product/2
  Product/1 -> eta/1

== system festo_proiect/model2/Rezervor ==
  q : Inport
  Constant : Constant  Value=C
  Gain : Gain  Gain=1/A
  Integrator : Integrator  InitialCondition=hinitial
  Product : Product
  Product1 : Product
  Scope : Scope
  Sqrt : Sqrt
  Sum : Sum  Inputs=|+-
  Sum1 : Sum  Inputs=|++
  step : Step  Commented=on  Time=300  After=0  SampleTime=0
  h : Outport
  disturbance_out : Outport  Port=2
  wires:
  q/1 -> Sum/1
  Sum/1 -> Gain/1
  Gain/1 -> Integrator/1
  Integrator/1 -> Sqrt/1, h/1
  Sqrt/1 -> Product1/1, Product/1
  Product/1 -> Sum/2, Scope/1  "qe"
  step/1 -> Sum1/2, Product1/2
  Constant/1 -> Sum1/1
  Sum1/1 -> Product/2
  Product1/1 -> disturbance_out/1

== system festo_proiect/model3/Amplificator ==
  ua : Inport
  Constant : Constant  Value=8.1
  Gain : Gain  Gain=2.2
  Gain1 : Gain  Gain=2.2
  Gain2 : Gain  Gain=5
  Saturation : Saturate  UpperLimit=22  LowerLimit=0
  Sum : Sum  Inputs=|++
  Sum1 : Sum  Inputs=|+-
  Switch : Switch  Threshold=8.1  SaturateOnIntegerOverflow=off  InputSameDT=off
  um : Outport
  wires:
  Sum/1 -> Switch/1
  Gain/1 -> Switch/3
  Saturation/1 -> um/1
  Switch/1 -> Saturation/1
  Sum1/1 -> Gain2/1
  Constant/1 -> Sum1/2
  Gain1/1 -> Sum/1
  ua/1 -> Gain1/1, Sum1/1, Gain/1, Switch/2
  Gain2/1 -> Sum/2

== system festo_proiect/model3/Curent rotoric ==
  q : Inport
  eta : Inport  Port=2
  h : Inport  Port=3
  um : Inport  Port=4
  "  " : Constant  Value=0.001
  Add : Sum  Inputs=|++
  Add1 : Sum  Inputs=|++
  Divide : Product  Inputs=**/
  Gain : Gain  Gain=2
  Gain1 : Gain  Gain=k
  Gain2 : Gain  Gain=1e4
  Product : Product
  Product1 : Product
  im : Outport
  wires:
  Gain1/1 -> Product/1
  Gain2/1 -> Product1/1
  eta/1 -> Gain2/1
  Divide/1 -> im/1
  Add1/1 -> Divide/3
  Add/1 -> Divide/1
  Product1/1 -> Add1/2
  "  "/1 -> Add1/1
  um/1 -> Product1/2
  Product/1 -> Add/2
  Gain/1 -> Add/1
  q/1 -> Product/2, Gain1/1, Divide/2
  h/1 -> Gain/1

== system festo_proiect/model3/Filtru ==
  q : Inport
  Integrator : Integrator  InitialCondition=qinitial
  Sum : Sum  Inputs=|+-
  q_f : Outport
  wires:
  Integrator/1 -> q_f/1, Sum/2
  Sum/1 -> Integrator/1
  q/1 -> Sum/1

== system festo_proiect/model3/Motor ==
  um : Inport
  im : Inport  Port=2
  Add : Sum  Inputs=+-
  Rm : Gain  Gain=3
  km*n : Outport
  wires:
  Add/1 -> km*n/1
  Rm/1 -> Add/2
  im/1 -> Rm/1
  um/1 -> Add/1

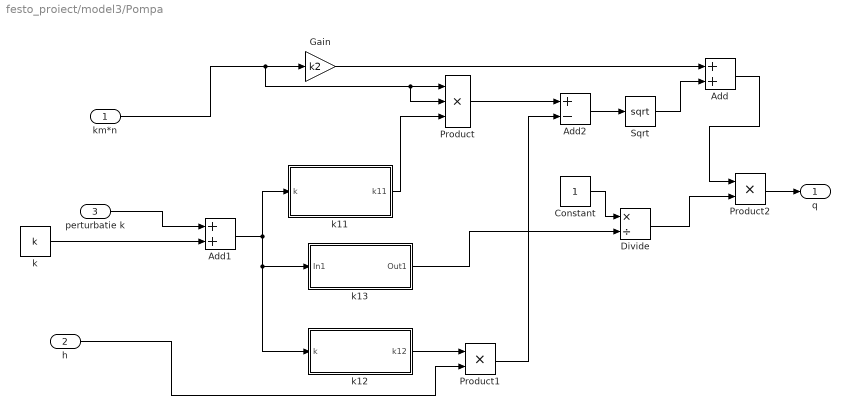
== system festo_proiect/model3/Pompa ==
  km*n : Inport
  h : Inport  Port=2
  perturbatie k : Inport  Port=3
  Add : Sum
  Add1 : Sum
  Add2 : Sum  Inputs=+-
  Constant : Constant
  Divide : Product  Inputs=*/
  Gain : Gain  Gain=k2
  Product : Product  Inputs=3
  Product1 : Product
  Product2 : Product
  Sqrt : Sqrt
  k : Constant  Value=k
  k11 : Subsystem
  k12 : Subsystem
  k13 : Subsystem
  q : Outport
  wires:
  Product2/1 -> q/1
  Divide/1 -> Product2/2
  Constant/1 -> Divide/1
  k13/1(Out1) -> Divide/2
  Add/1 -> Product2/1
  Sqrt/1 -> Add/2
  Add2/1 -> Sqrt/1
  Product1/1 -> Add2/2
  k12/1(k12) -> Product1/1
  h/1 -> Product1/2
  Product/1 -> Add2/1
  Gain/1 -> Add/1
  k11/1(k11) -> Product/3
  Add1/1 -> k13/1(In1), k12/1(k), k11/1(k)
  k/1 -> Add1/2
  perturbatie k/1 -> Add1/1
  km*n/1 -> Gain/1, Product/1, Product/2

== system festo_proiect/model3/Randament pompa ==
  q : Inport
  um : Inport  Port=2
  Gain : Gain  Gain=keta
  Product : Product
  eta : Outport
  wires:
  Product/1 -> eta/1
  Gain/1 -> Product/2
  q/1 -> Product/1
  um/1 -> Gain/1

== system festo_proiect/model3/Rezervor ==
  q : Inport
  Constant : Constant  Value=C
  Gain : Gain  Gain=1/A
  Integrator : Integrator  InitialCondition=hinitial
  Product : Product
  Product1 : Product
  Scope : Scope
  Sqrt : Sqrt
  Sum : Sum  Inputs=|+-
  Sum1 : Sum  Inputs=|++
  step : Step  Time=300  After=2  SampleTime=0
  h : Outport
  disturbance_out : Outport  Port=2
  wires:
  Product1/1 -> disturbance_out/1
  Sum1/1 -> Product/2
  Constant/1 -> Sum1/1
  step/1 -> Product1/2, Sum1/2
  Product/1 -> Scope/1, Sum/2  "qe"
  Sqrt/1 -> Product/1, Product1/1
  Integrator/1 -> h/1, Sqrt/1
  Gain/1 -> Integrator/1
  Sum/1 -> Gain/1
  q/1 -> Sum/1

== system festo_proiect/model4/Amplificator ==
  ua : Inport
  Constant : Constant  Value=8.1
  Gain : Gain  Gain=2.2
  Gain1 : Gain  Gain=2.2
  Gain2 : Gain  Gain=5
  Saturation : Saturate  UpperLimit=22  LowerLimit=0
  Sum : Sum  Inputs=|++
  Sum1 : Sum  Inputs=|+-
  Switch : Switch  Threshold=8.1  SaturateOnIntegerOverflow=off  InputSameDT=off
  um : Outport
  wires:
  Gain2/1 -> Sum/2
  ua/1 -> Switch/2, Gain/1, Sum1/1, Gain1/1
  Gain1/1 -> Sum/1
  Constant/1 -> Sum1/2
  Sum1/1 -> Gain2/1
  Switch/1 -> Saturation/1
  Saturation/1 -> um/1
  Gain/1 -> Switch/3
  Sum/1 -> Switch/1

== system festo_proiect/model4/Curent rotoric ==
  q : Inport
  eta : Inport  Port=2
  h : Inport  Port=3
  um : Inport  Port=4
  "  " : Constant  Value=0.001
  Add : Sum  Inputs=|++
  Add1 : Sum  Inputs=|++
  Divide : Product  Inputs=**/
  Gain : Gain  Gain=2
  Gain1 : Gain  Gain=k
  Gain2 : Gain  Gain=1e4
  Product : Product
  Product1 : Product
  im : Outport
  wires:
  h/1 -> Gain/1
  q/1 -> Divide/2, Gain1/1, Product/2
  Gain/1 -> Add/1
  Product/1 -> Add/2
  um/1 -> Product1/2
  "  "/1 -> Add1/1
  Product1/1 -> Add1/2
  Add/1 -> Divide/1
  Add1/1 -> Divide/3
  Divide/1 -> im/1
  eta/1 -> Gain2/1
  Gain2/1 -> Product1/1
  Gain1/1 -> Product/1

== system festo_proiect/model4/Filtru ==
  q : Inport
  Integrator : Integrator  InitialCondition=qinitial
  Sum : Sum  Inputs=|+-
  q_f : Outport
  wires:
  q/1 -> Sum/1
  Sum/1 -> Integrator/1
  Integrator/1 -> Sum/2, q_f/1

== system festo_proiect/model4/Motor ==
  um : Inport
  im : Inport  Port=2
  Add : Sum  Inputs=+-
  Rm : Gain  Gain=3
  km*n : Outport
  wires:
  um/1 -> Add/1
  im/1 -> Rm/1
  Rm/1 -> Add/2
  Add/1 -> km*n/1

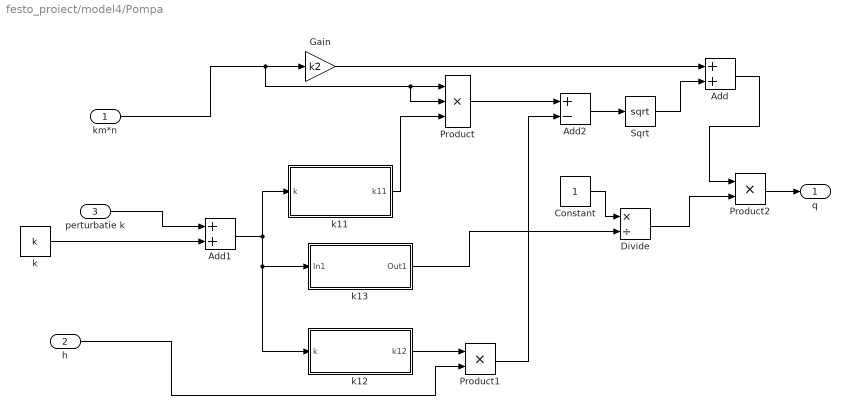
== system festo_proiect/model4/Pompa ==
  km*n : Inport
  h : Inport  Port=2
  perturbatie k : Inport  Port=3
  Add : Sum
  Add1 : Sum
  Add2 : Sum  Inputs=+-
  Constant : Constant
  Divide : Product  Inputs=*/
  Gain : Gain  Gain=k2
  Product : Product  Inputs=3
  Product1 : Product
  Product2 : Product
  Sqrt : Sqrt
  k : Constant  Value=k
  k11 : Subsystem
  k12 : Subsystem
  k13 : Subsystem
  q : Outport
  wires:
  km*n/1 -> Product/2, Product/1, Gain/1
  perturbatie k/1 -> Add1/1
  k/1 -> Add1/2
  Add1/1 -> k11/1(k), k12/1(k), k13/1(In1)
  k11/1(k11) -> Product/3
  Gain/1 -> Add/1
  Product/1 -> Add2/1
  h/1 -> Product1/2
  k12/1(k12) -> Product1/1
  Product1/1 -> Add2/2
  Add2/1 -> Sqrt/1
  Sqrt/1 -> Add/2
  Add/1 -> Product2/1
  k13/1(Out1) -> Divide/2
  Constant/1 -> Divide/1
  Divide/1 -> Product2/2
  Product2/1 -> q/1

== system festo_proiect/model4/Randament pompa ==
  q : Inport
  um : Inport  Port=2
  Gain : Gain  Gain=keta
  Product : Product
  eta : Outport
  wires:
  um/1 -> Gain/1
  q/1 -> Product/1
  Gain/1 -> Product/2
  Product/1 -> eta/1

== system festo_proiect/model4/Rezervor ==
  q : Inport
  Constant : Constant  Value=C
  Gain : Gain  Gain=1/A
  Integrator : Integrator  InitialCondition=hinitial
  Product : Product
  Product1 : Product
  Scope : Scope
  Sqrt : Sqrt
  Sum : Sum  Inputs=|+-
  Sum1 : Sum  Inputs=|++
  step : Step  Commented=on  Time=300  After=2  SampleTime=0
  h : Outport
  disturbance_out : Outport  Port=2
  wires:
  q/1 -> Sum/1
  Sum/1 -> Gain/1
  Gain/1 -> Integrator/1
  Integrator/1 -> Sqrt/1, h/1
  Sqrt/1 -> Product1/1, Product/1
  Product/1 -> Sum/2, Scope/1  "qe"
  step/1 -> Sum1/2, Product1/2
  Constant/1 -> Sum1/1
  Sum1/1 -> Product/2
  Product1/1 -> disturbance_out/1

== system festo_proiect/model5/Amplificator ==
  ua : Inport
  Constant : Constant  Value=8.1
  Gain : Gain  Gain=2.2
  Gain1 : Gain  Gain=2.2
  Gain2 : Gain  Gain=5
  Saturation : Saturate  UpperLimit=22  LowerLimit=0
  Sum : Sum  Inputs=|++
  Sum1 : Sum  Inputs=|+-
  Switch : Switch  Threshold=8.1  SaturateOnIntegerOverflow=off  InputSameDT=off
  um : Outport
  wires:
  Sum/1 -> Switch/1
  Gain/1 -> Switch/3
  Saturation/1 -> um/1
  Switch/1 -> Saturation/1
  Sum1/1 -> Gain2/1
  Constant/1 -> Sum1/2
  Gain1/1 -> Sum/1
  ua/1 -> Gain1/1, Sum1/1, Gain/1, Switch/2
  Gain2/1 -> Sum/2

== system festo_proiect/model5/Curent rotoric ==
  q : Inport
  eta : Inport  Port=2
  h : Inport  Port=3
  um : Inport  Port=4
  "  " : Constant  Value=0.001
  Add : Sum  Inputs=|++
  Add1 : Sum  Inputs=|++
  Divide : Product  Inputs=**/
  Gain : Gain  Gain=2
  Gain1 : Gain  Gain=k
  Gain2 : Gain  Gain=1e4
  Product : Product
  Product1 : Product
  im : Outport
  wires:
  Gain1/1 -> Product/1
  Gain2/1 -> Product1/1
  eta/1 -> Gain2/1
  Divide/1 -> im/1
  Add1/1 -> Divide/3
  Add/1 -> Divide/1
  Product1/1 -> Add1/2
  "  "/1 -> Add1/1
  um/1 -> Product1/2
  Product/1 -> Add/2
  Gain/1 -> Add/1
  q/1 -> Product/2, Gain1/1, Divide/2
  h/1 -> Gain/1

== system festo_proiect/model5/Filtru ==
  q : Inport
  Integrator : Integrator  InitialCondition=qinitial
  Sum : Sum  Inputs=|+-
  q_f : Outport
  wires:
  Integrator/1 -> q_f/1, Sum/2
  Sum/1 -> Integrator/1
  q/1 -> Sum/1
